simulink model "parteIX"  (R2018a)
settings: Solver=VariableStepAuto  StartTime=0.0  StopTime=10.0  RelTol=1e-3
values from neighbouring files (symbols this model uses):
  A_0 = [0 -3.26931291643 0 0.71460251427 0 0 0 0 1 -0.0325743287495 0 -0.000548520916999 ... (64 elements, 8x8)]    [parametros.mat]    (also in twin_rotor_modelo_V1.m = eval(A_0))
  B_0 = [0 0 0 0 0 0 1190.47619048 0 0 0 0 0 ... (16 elements, 8x2)]    [parametros.mat]    (also in twin_rotor_modelo_V1.m = eval(B_0))
  C_0 = [1 0 0 0 0 1 0 0 0 0 0 0 ... (16 elements, 2x8)]    [parametros.mat]    (also in twin_rotor_modelo_V1.m = eval(C_0))
  D_0 = [0  0; 0  0]    [parametros.mat]    (also in twin_rotor_modelo_V1.m = eval(D_0))
  Q = [ ... (first row only)    [ele_cu_erre_para_iterar.m]    (also in elecuerre.m)
  R = [ ... (first row only)    [ele_cu_erre_para_iterar.m]    (also in elecuerre.m; twin_rotor_modelo_V1.m = R2*R1)
  u0 = [11.9668031953 -0.0853053139382]    [parametros.mat]    (also in twin_rotor_modelo_V1.m = [u_p_0;u_t_0])
undefined symbols (not defined in the file or in its folder): K
settings Model: Creator=Gonzalo  LastModifiedBy=Gonzalo

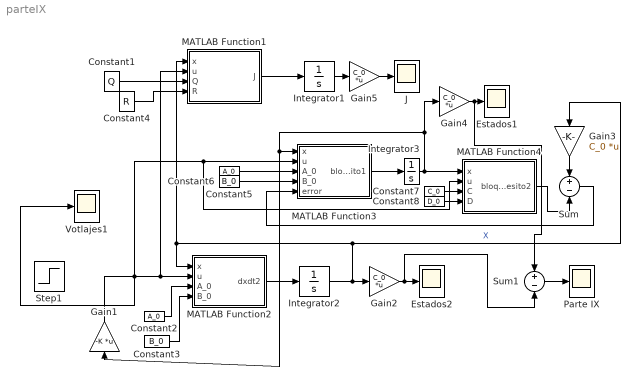
== system parteIX ==
  Constant1 : Constant  Value=Q
  Constant2 : Constant  Value=A_0
  Constant3 : Constant  Value=B_0
  Constant4 : Constant  Value=R
  Constant5 : Constant  Value=A_0
  Constant6 : Constant  Value=B_0
  Constant7 : Constant  Value=C_0
  Constant8 : Constant  Value=D_0
  Estados1 : Scope
  Estados2 : Scope
  Gain1 : Gain  Gain=-K  Multiplication=Matrix(K*u)
  Gain{2..5} (4 alike) : Gain  Gain=C_0  Multiplication=Matrix(K*u)
  Integrator1 : Integrator  InitialCondition=[pi/6 0 0 0 0 0 0 0]
  Integrator2 : Integrator  InitialCondition=[pi/6 0 0 0 0 0 0 0]
  Integrator3 : Integrator  InitialCondition=[pi/6 0 0 0 0 0 0 0]
  J : Scope
  MATLAB Function1 : MATLAB Function  TreatAsAtomicUnit=on
  MATLAB Function2 : MATLAB Function  TreatAsAtomicUnit=on
  MATLAB Function3 : MATLAB Function  TreatAsAtomicUnit=on
  MATLAB Function4 : MATLAB Function  TreatAsAtomicUnit=on
  Parte IX : Scope
  Step1 : Step  Time=10  Before=u0  After=u0  SampleTime=0
  Sum : Sum  Inputs=+|-
  Sum1 : Sum  Inputs=+|-
  Votlajes1 : Scope
  wires:
  Integrator3/1 -> MATLAB Function4/1(x), Gain4/1, MATLAB Function3/1(x), Gain1/1
  Gain3/1 -> Sum/1
  MATLAB Function4/1(bloquesito2) -> Sum/2
  Gain4/1 -> Sum1/1, Estados1/1
  Constant4/1 -> MATLAB Function1/4(R)
  Constant1/1 -> MATLAB Function1/3(Q)
  Integrator2/1 -> Gain3/1, MATLAB Function1/1(x), MATLAB Function2/1(x), Gain2/1  "X"
  Constant5/1 -> MATLAB Function3/3(A_0)
  Constant2/1 -> MATLAB Function2/3(A_0)
  MATLAB Function3/1(bloquesito1) -> Integrator3/1
  Constant8/1 -> MATLAB Function4/4(D)
  Constant7/1 -> MATLAB Function4/3(C)
  Constant6/1 -> MATLAB Function3/4(B_0)
  MATLAB Function2/1(dxdt2) -> Integrator2/1
  Gain2/1 -> Sum1/2, Estados2/1
  Sum1/1 -> Parte IX/1
  MATLAB Function1/1(J) -> Integrator1/1
  Gain1/1 -> Votlajes1/1, MATLAB Function2/2(u), MATLAB Function1/2(u), MATLAB Function3/2(u), MATLAB Function4/2(u)
  Constant3/1 -> MATLAB Function2/4(B_0)
  Sum/1 -> MATLAB Function3/5(error)
  Integrator1/1 -> Gain5/1
  Gain5/1 -> J/1

== matlab function parteIX/MATLAB Function1 ==
  data: x input; u input; J output; Q input; R input
function J = funcion(x,u,Q,R)
J = x'*Q*x + u'*R*u;

== matlab function parteIX/MATLAB Function3 ==
  data: x input; u input; bloquesito1 output; A_0 input; B_0 input; error input
function bloquesito1 = funcion(x,u,A_0,B_0, error)
L =[
    0.0187   -0.0107;
   -0.0006   -0.0012;
   -0.0037    0.0796;
    0.0001    0.0004;
   -0.0000    0.0000;
    0.0000   -0.0000;
    0.0000   -0.0000;
    0.0000    0.0000];
bloquesito1 = A_0*x + B_0*u + L*error

== matlab function parteIX/MATLAB Function2 ==
  data: x input; u input; dxdt2 output; A_0 input; B_0 input
function dxdt2 = funcion(x,u,A_0,B_0)
dxdt2 = A_0*x + B_0*u;

== matlab function parteIX/MATLAB Function4 ==
  data: x input; u input; bloquesito2 output; C input; D input
function bloquesito2 = funcion(x,u,C,D)
bloquesito2 = C*x + D*u
